simulink model "simulink_E6"  (R2024a)
settings: Solver=VariableStepAuto  StartTime=0.0  StopTime=10.0  RelTol=1e-3
values from neighbouring files (symbols this model uses):
  a = K(3)    [E6_fobj.m]
  K1 = K(1)    [E6_fobj.m]
  K2 = K(2)    [E6_fobj.m]
  x0 = [0 3]'    [E6_fobj.m]
  y0 = 10    [E6_fobj.m]
settings Model: Creator=claudio  LastModifiedBy=stefa
settings SolverCC: AlgebraicLoopSolver=TrustRegion
settings DataIOCC: ReturnWorkspaceOutputs=off
settings DebuggingCC: UnconnectedInputMsg=warning  UnconnectedOutputMsg=warning  UnconnectedLineMsg=warning  ArithmeticOperatorsInVariantConditions=warning
settings ModelReferenceCC: EnableRefExpFcnMdlSchedulingChecks=on
settings SFSimCC: SimUseLocalCustomCode=off  CustomCodeUndefinedFunction=UseInterfaceOnly
settings RTWCC: RTWUseLocalCustomCode=off  GPUComputeCapability=3.5

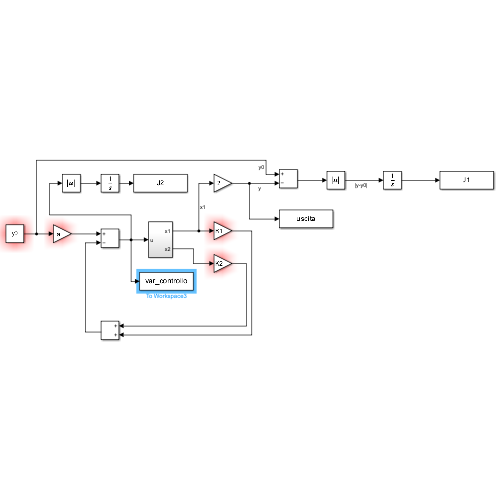
[thumbnail: Simulink's stored preview of the top-level diagram]
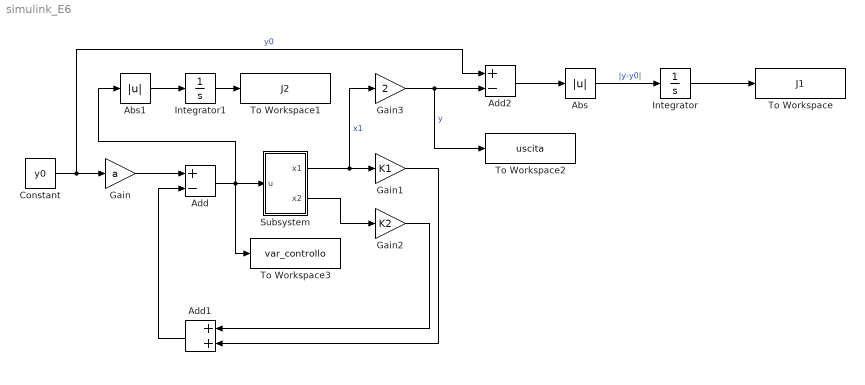
== system simulink_E6 ==
  Abs : Abs  SaturateOnIntegerOverflow=off
  Abs1 : Abs  SaturateOnIntegerOverflow=off
  Add : Sum  Inputs=+-
  Add1 : Sum
  Add2 : Sum  Inputs=+-
  Constant : Constant  Value=y0
  Gain : Gain  Gain=a
  Gain1 : Gain  Gain=K1
  Gain2 : Gain  Gain=K2
  Gain3 : Gain  Gain=2
  Integrator : Integrator
  Integrator1 : Integrator
  Subsystem : Subsystem
  To Workspace : ToWorkspace  VariableName=J1  SampleTime=-1
  To Workspace1 : ToWorkspace  VariableName=J2  SampleTime=-1
  To Workspace2 : ToWorkspace  VariableName=uscita  SaveFormat=Structure With Time  SampleTime=-1
  To Workspace3 : ToWorkspace  VariableName=var_controllo  SaveFormat=Structure With Time  SampleTime=-1
  wires:
  Add/1 -> To Workspace3/1, Abs1/1, Subsystem/1(u)
  Constant/1 -> Add2/1, Gain/1  "y0"
  Gain/1 -> Add/1
  Subsystem/1(x1) -> Gain3/1, Gain1/1  "x1"
  Subsystem/2(x2) -> Gain2/1
  Gain2/1 -> Add1/1
  Gain1/1 -> Add1/2
  Add1/1 -> Add/2
  Gain3/1 -> To Workspace2/1, Add2/2  "y"
  Add2/1 -> Abs/1
  Abs/1 -> Integrator/1  "|y-y0|"
  Abs1/1 -> Integrator1/1
  Integrator/1 -> To Workspace/1
  Integrator1/1 -> To Workspace1/1

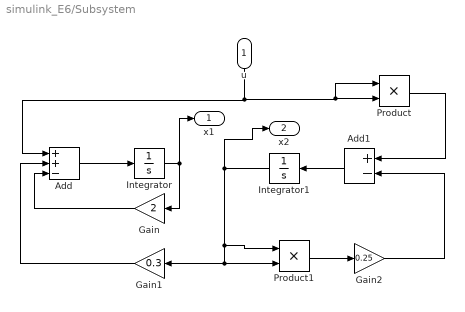
== system simulink_E6/Subsystem ==
  u : Inport
  Add : Sum  Inputs=++-
  Add1 : Sum  Inputs=+-
  Gain : Gain  Gain=2
  Gain1 : Gain  Gain=0.3
  Gain2 : Gain  Gain=0.25
  Integrator : Integrator  InitialCondition=x0(1)  LimitOutput=on  UpperSaturationLimit=1000  LowerSaturationLimit=-1000
  Integrator1 : Integrator  InitialCondition=x0(2)  LimitOutput=on  UpperSaturationLimit=1000  LowerSaturationLimit=-1000
  Product : Product
  Product1 : Product
  x1 : Outport  VectorParamsAs1DForOutWhenUnconnected=off
  x2 : Outport  Port=2  VectorParamsAs1DForOutWhenUnconnected=off
  wires:
  Add/1 -> Integrator/1
  Product1/1 -> Gain2/1
  Gain/1 -> Add/3
  Integrator/1 -> x1/1, Gain/1
  u/1 -> Product/2, Product/1, Add/1
  Gain1/1 -> Add/2
  Gain2/1 -> Add1/2
  Add1/1 -> Integrator1/1
  Product/1 -> Add1/1
  Integrator1/1 -> x2/1, Product1/1, Product1/2, Gain1/1
